simulink model "understandingof_cosecwave"  (R2024b)
settings: Solver=VariableStepAuto  StartTime=0.0  StopTime=10.0  MaxStep=0.001  RelTol=1e-3
settings Model: Creator=admin  LastModifiedBy=admin

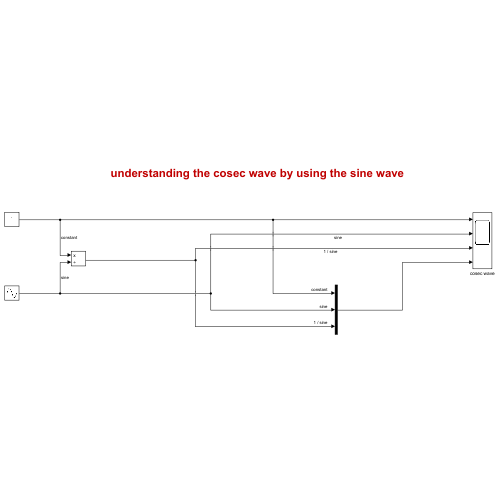
[thumbnail: Simulink's stored preview of the top-level diagram]
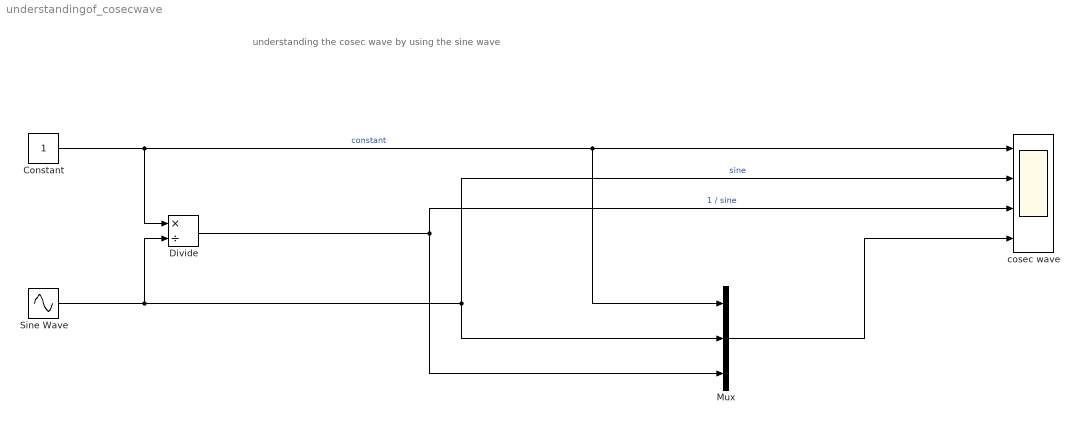
== system understandingof_cosecwave ==
  note: understanding the cosec wave by using the sine wave
  Constant : Constant
  Divide : Product  Inputs=*/
  Mux : Mux  Inputs=3
  Sine Wave : Sin  SampleTime=0
  cosec wave : Scope  NumInputPorts=4
  wires:
  Constant/1 -> Mux/1, cosec wave/1, Divide/1  "constant"
  Sine Wave/1 -> cosec wave/2, Mux/2, Divide/2  "sine"
  Divide/1 -> cosec wave/3, Mux/3  "1 / sine"
  Mux/1 -> cosec wave/4
